simulink model "generator_trajektorie"  (R2020a)
settings: Solver=VariableStepAuto  StartTime=0.0  StopTime=Tmax  RelTol=1e-3
values from neighbouring files (symbols this model uses):
  a1 = 2    [overeniFunkcionality.m]    (also in pohyb_po_trajektorii.m; setup.m)
  a2 = 1.5    [overeniFunkcionality.m]    (also in pohyb_po_trajektorii.m; setup.m)
  a3 = 0.5    [overeniFunkcionality.m]    (also in pohyb_po_trajektorii.m; setup.m)
  r = a1-a2-a3    (= 0)    [overeniFunkcionality.m]    (also in pohyb_po_trajektorii.m; setup.m)
  R = a1+a2+a3    (= 4)    [overeniFunkcionality.m]    (also in pohyb_po_trajektorii.m; setup.m)
  T_1_0 = [cos(theta10), -sin(theta10), 0, a1*cos(theta10) ... (first row only)    [overeniFunkcionality.m]    (also in pohyb_po_trajektorii.m; setup.m)
  T_2_1 = [cos(theta20), -sin(theta20), 0, a2*cos(theta20) ... (first row only)    [overeniFunkcionality.m]    (also in pohyb_po_trajektorii.m; setup.m)
  T_3_2 = [cos(theta30), -sin(theta30), 0, a3*cos(theta30) ... (first row only)    [overeniFunkcionality.m]    (also in pohyb_po_trajektorii.m; setup.m)
  v = 0.5    [overeniFunkcionality.m]    (also in pohyb_po_trajektorii.m; setup.m)
  vmax = 1    [pohyb_po_trajektorii.m]
undefined symbols (not defined in the file or in its folder): X, Y, Z
libraries: sm_lib x56, nesl_utility x32
(part 2 of 2)

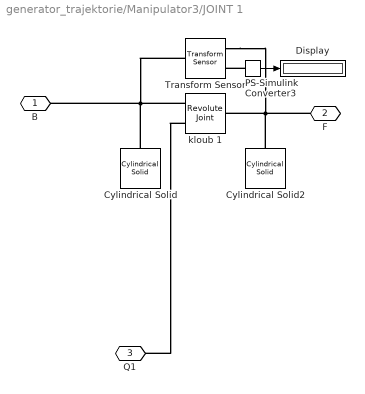
== system generator_trajektorie/Manipulator3/JOINT 1 ==
  Cylindrical Solid : sm_lib/Body Elements/Cylindrical Solid  GraphicAmbientColor=[0.15 0.15 0.15 1.0]  BasedOnType=Density  CenterOfMass=[0 0 0]  CenterOfMassUnits=m  GraphicDiffuseColor=[0.5 0.5 0.5]  CylinderLength=0.1  CylinderLengthUnits=m  CylinderRadius=0.05  CylinderRadiusUnits=m  Density=1000  DensityUnits=kg/m^3  DoExposeReferenceFrame=on  GraphicEmissiveColor=[0.0 0.0 0.0 1.0]  ExportEntireGeometry=off  SerializedFrames=<Frames/>  MarkerShape=Sphere  MarkerSize=10  GraphicType=FromGeometry  InertiaType=CalculateFromGeometry  Mass=1  MassUnits=kg  MomentsOfInertia=[1 1 1]  MomentsOfInertiaUnits=kg*m^2  GraphicOpacity=1.0  ProductsOfInertia=[0 0 0]  ProductsOfInertiaUnits=kg*m^2  GraphicShininess=75  GraphicSpecularColor=[0.5 0.5 0.5 1.0]  GraphicVisPropType=SimpleVisualProperties
  Cylindrical Solid2 : sm_lib/Body Elements/Cylindrical Solid  GraphicAmbientColor=[0.15 0.15 0.15 1.0]  BasedOnType=Density  CenterOfMass=[0 0 0]  CenterOfMassUnits=m  GraphicDiffuseColor=[0.5 0.5 0.5]  CylinderLength=0.05  CylinderLengthUnits=m  CylinderRadius=0.1  CylinderRadiusUnits=m  Density=1000  DensityUnits=kg/m^3  DoExposeReferenceFrame=on  GraphicEmissiveColor=[0.0 0.0 0.0 1.0]  ExportEntireGeometry=off  SerializedFrames=<Frames/>  MarkerShape=Sphere  MarkerSize=10  GraphicType=FromGeometry  InertiaType=CalculateFromGeometry  Mass=1  MassUnits=kg  MomentsOfInertia=[1 1 1]  MomentsOfInertiaUnits=kg*m^2  GraphicOpacity=1.0  ProductsOfInertia=[0 0 0]  ProductsOfInertiaUnits=kg*m^2  GraphicShininess=75  GraphicSpecularColor=[0.5 0.5 0.5 1.0]  GraphicVisPropType=SimpleVisualProperties
  Display : Display
  PS-Simulink Converter3 : nesl_utility/PS-Simulink Converter  PhysicalDomain=network_engine_domain  SubClassName=ps_output  LeftPortType=input  RightPortType=output  PseudoPeriodic=off  Frequencies=[]  Unit=inherit  AffineConversion=off
  Transform Sensor : sm_lib/Frames and Transforms/Transform Sensor  MeasurementFrame=Base  SenseAngle=on  SenseAxis=off  SenseAngle1=off  SenseAngle2=off  SenseAngle3=off  SenseQ=off  SenseR=off  SenseOmegaX=off  SenseOmegaY=off  SenseOmegaZ=off  SenseOmega1=off  SenseOmega2=off  SenseOmega3=off  SenseQDot=off  SenseRDot=off  SenseAlphaX=off  SenseAlphaY=off  SenseAlphaZ=off  SenseAlpha1=off  SenseAlpha2=off  SenseAlpha3=off  SenseQDDot=off  SenseRDDot=off  SenseX=off  SenseY=off  SenseZ=off  SenseRad=off  SenseAzim=off  SenseDist=off  SenseInc=off  SenseXDot=off  SenseYDot=off  SenseZDot=off  SenseRadDot=off  SenseAzimDot=off  SenseDistDot=off  SenseIncDot=off  SenseXDDot=off  SenseYDDot=off  SenseZDDot=off  SenseRadDDot=off  SenseAzimDDot=off  SenseDistDDot=off  SenseIncDDot=off
  kloub 1 : sm_lib/Joints/Revolute Joint  JointMode=Normal  SenseConstraintForce=off  SenseConstraintForceX=off  SenseConstraintForceY=off  SenseConstraintForceZ=off  SenseConstraintTorque=off  SenseConstraintTorqueX=off  SenseConstraintTorqueY=off  SenseConstraintTorqueZ=off  SenseTotalForce=off  SenseTotalForceX=off  SenseTotalForceY=off  SenseTotalForceZ=off  SenseTotalTorque=off  SenseTotalTorqueX=off  SenseTotalTorqueY=off  SenseTotalTorqueZ=off  CompositeWrenchDir=FollowerOnBase  CompositeWrenchFrame=BaseFrame  EquilibriumPosition=0  EquilibriumPositionUnits=deg  SpringStiffness=0  SpringStiffnessUnits=N*m/deg  DampingCoefficient=0  DampingCoefficientUnits=N*m/(deg/s)  TorqueActuationMode=ComputedTorque  MotionActuationMode=InputMotion  SensePosition=off  SenseVelocity=off  SenseAcceleration=off  SenseTorqueForce=off  SenseLowerLimitTorqueForce=off  SenseUpperLimitTorqueForce=off  LowerLimitSpecify=off  LowerLimitBound=-90  LowerLimitBoundUnits=deg  LowerLimitStiffness=1e4  LowerLimitStiffnessUnits=N*m/deg  LowerLimitDamping=10  LowerLimitDampingUnits=N*m/(deg/s)  LowerLimitTransitionRegionWidth=0.1  LowerLimitTransitionRegionWidthUnits=deg  UpperLimitSpecify=off  UpperLimitBound=90  UpperLimitBoundUnits=deg  UpperLimitStiffness=1e4  UpperLimitStiffnessUnits=N*m/deg  UpperLimitDamping=10  UpperLimitDampingUnits=N*m/(deg/s)  UpperLimitTransitionRegionWidth=0.1  UpperLimitTransitionRegionWidthUnits=deg  PositionTargetSpecify=off  PositionTargetPriority=High  PositionTargetValue=0  PositionTargetValueUnits=deg  VelocityTargetSpecify=off  VelocityTargetPriority=High  VelocityTargetValue=0  VelocityTargetValueUnits=deg/s
  B : PMIOPort  Side=Left
  F : PMIOPort  Port=2  Side=Right
  Q1 : PMIOPort  Port=3  Side=Left
  wires:
  PS-Simulink Converter3/1 -> Display/1
  connections:
  Cylindrical Solid2/RConn1 -- F/RConn1 -- Transform Sensor/RConn1 -- kloub 1/RConn1
  Transform Sensor/LConn1 -- B/RConn1 -- kloub 1/LConn1 -- Cylindrical Solid/RConn1
  PS-Simulink Converter3/LConn1 -- Transform Sensor/RConn2
  kloub 1/LConn2 -- Q1/RConn1

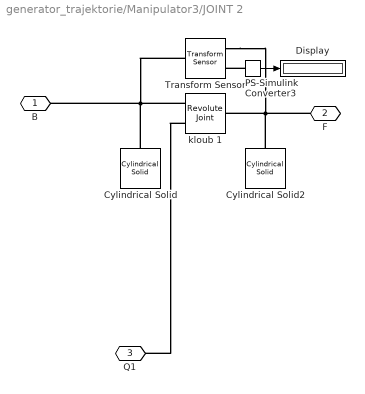
== system generator_trajektorie/Manipulator3/JOINT 2 ==
  Cylindrical Solid : sm_lib/Body Elements/Cylindrical Solid  GraphicAmbientColor=[0.15 0.15 0.15 1.0]  BasedOnType=Density  CenterOfMass=[0 0 0]  CenterOfMassUnits=m  GraphicDiffuseColor=[0.5 0.5 0.5]  CylinderLength=0.1  CylinderLengthUnits=m  CylinderRadius=0.05  CylinderRadiusUnits=m  Density=1000  DensityUnits=kg/m^3  DoExposeReferenceFrame=on  GraphicEmissiveColor=[0.0 0.0 0.0 1.0]  ExportEntireGeometry=off  SerializedFrames=<Frames/>  MarkerShape=Sphere  MarkerSize=10  GraphicType=FromGeometry  InertiaType=CalculateFromGeometry  Mass=1  MassUnits=kg  MomentsOfInertia=[1 1 1]  MomentsOfInertiaUnits=kg*m^2  GraphicOpacity=1.0  ProductsOfInertia=[0 0 0]  ProductsOfInertiaUnits=kg*m^2  GraphicShininess=75  GraphicSpecularColor=[0.5 0.5 0.5 1.0]  GraphicVisPropType=SimpleVisualProperties
  Cylindrical Solid2 : sm_lib/Body Elements/Cylindrical Solid  GraphicAmbientColor=[0.15 0.15 0.15 1.0]  BasedOnType=Density  CenterOfMass=[0 0 0]  CenterOfMassUnits=m  GraphicDiffuseColor=[0.5 0.5 0.5]  CylinderLength=0.05  CylinderLengthUnits=m  CylinderRadius=0.1  CylinderRadiusUnits=m  Density=1000  DensityUnits=kg/m^3  DoExposeReferenceFrame=on  GraphicEmissiveColor=[0.0 0.0 0.0 1.0]  ExportEntireGeometry=off  SerializedFrames=<Frames/>  MarkerShape=Sphere  MarkerSize=10  GraphicType=FromGeometry  InertiaType=CalculateFromGeometry  Mass=1  MassUnits=kg  MomentsOfInertia=[1 1 1]  MomentsOfInertiaUnits=kg*m^2  GraphicOpacity=1.0  ProductsOfInertia=[0 0 0]  ProductsOfInertiaUnits=kg*m^2  GraphicShininess=75  GraphicSpecularColor=[0.5 0.5 0.5 1.0]  GraphicVisPropType=SimpleVisualProperties
  Display : Display
  PS-Simulink Converter3 : nesl_utility/PS-Simulink Converter  PhysicalDomain=network_engine_domain  SubClassName=ps_output  LeftPortType=input  RightPortType=output  PseudoPeriodic=off  Frequencies=[]  Unit=inherit  AffineConversion=off
  Transform Sensor : sm_lib/Frames and Transforms/Transform Sensor  MeasurementFrame=Base  SenseAngle=on  SenseAxis=off  SenseAngle1=off  SenseAngle2=off  SenseAngle3=off  SenseQ=off  SenseR=off  SenseOmegaX=off  SenseOmegaY=off  SenseOmegaZ=off  SenseOmega1=off  SenseOmega2=off  SenseOmega3=off  SenseQDot=off  SenseRDot=off  SenseAlphaX=off  SenseAlphaY=off  SenseAlphaZ=off  SenseAlpha1=off  SenseAlpha2=off  SenseAlpha3=off  SenseQDDot=off  SenseRDDot=off  SenseX=off  SenseY=off  SenseZ=off  SenseRad=off  SenseAzim=off  SenseDist=off  SenseInc=off  SenseXDot=off  SenseYDot=off  SenseZDot=off  SenseRadDot=off  SenseAzimDot=off  SenseDistDot=off  SenseIncDot=off  SenseXDDot=off  SenseYDDot=off  SenseZDDot=off  SenseRadDDot=off  SenseAzimDDot=off  SenseDistDDot=off  SenseIncDDot=off
  kloub 1 : sm_lib/Joints/Revolute Joint  JointMode=Normal  SenseConstraintForce=off  SenseConstraintForceX=off  SenseConstraintForceY=off  SenseConstraintForceZ=off  SenseConstraintTorque=off  SenseConstraintTorqueX=off  SenseConstraintTorqueY=off  SenseConstraintTorqueZ=off  SenseTotalForce=off  SenseTotalForceX=off  SenseTotalForceY=off  SenseTotalForceZ=off  SenseTotalTorque=off  SenseTotalTorqueX=off  SenseTotalTorqueY=off  SenseTotalTorqueZ=off  CompositeWrenchDir=FollowerOnBase  CompositeWrenchFrame=BaseFrame  EquilibriumPosition=0  EquilibriumPositionUnits=deg  SpringStiffness=0  SpringStiffnessUnits=N*m/deg  DampingCoefficient=0  DampingCoefficientUnits=N*m/(deg/s)  TorqueActuationMode=ComputedTorque  MotionActuationMode=InputMotion  SensePosition=off  SenseVelocity=off  SenseAcceleration=off  SenseTorqueForce=off  SenseLowerLimitTorqueForce=off  SenseUpperLimitTorqueForce=off  LowerLimitSpecify=off  LowerLimitBound=-90  LowerLimitBoundUnits=deg  LowerLimitStiffness=1e4  LowerLimitStiffnessUnits=N*m/deg  LowerLimitDamping=10  LowerLimitDampingUnits=N*m/(deg/s)  LowerLimitTransitionRegionWidth=0.1  LowerLimitTransitionRegionWidthUnits=deg  UpperLimitSpecify=off  UpperLimitBound=90  UpperLimitBoundUnits=deg  UpperLimitStiffness=1e4  UpperLimitStiffnessUnits=N*m/deg  UpperLimitDamping=10  UpperLimitDampingUnits=N*m/(deg/s)  UpperLimitTransitionRegionWidth=0.1  UpperLimitTransitionRegionWidthUnits=deg  PositionTargetSpecify=off  PositionTargetPriority=High  PositionTargetValue=0  PositionTargetValueUnits=deg  VelocityTargetSpecify=off  VelocityTargetPriority=High  VelocityTargetValue=0  VelocityTargetValueUnits=deg/s
  B : PMIOPort  Side=Left
  F : PMIOPort  Port=2  Side=Right
  Q1 : PMIOPort  Port=3  Side=Left
  wires:
  PS-Simulink Converter3/1 -> Display/1
  connections:
  Transform Sensor/RConn1 -- Cylindrical Solid2/RConn1 -- kloub 1/RConn1 -- F/RConn1
  kloub 1/LConn1 -- Transform Sensor/LConn1 -- Cylindrical Solid/RConn1 -- B/RConn1
  PS-Simulink Converter3/LConn1 -- Transform Sensor/RConn2
  kloub 1/LConn2 -- Q1/RConn1

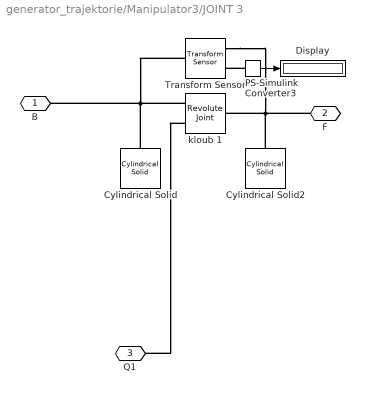
== system generator_trajektorie/Manipulator3/JOINT 3 ==
  Cylindrical Solid : sm_lib/Body Elements/Cylindrical Solid  GraphicAmbientColor=[0.15 0.15 0.15 1.0]  BasedOnType=Density  CenterOfMass=[0 0 0]  CenterOfMassUnits=m  GraphicDiffuseColor=[0.5 0.5 0.5]  CylinderLength=0.1  CylinderLengthUnits=m  CylinderRadius=0.05  CylinderRadiusUnits=m  Density=1000  DensityUnits=kg/m^3  DoExposeReferenceFrame=on  GraphicEmissiveColor=[0.0 0.0 0.0 1.0]  ExportEntireGeometry=off  SerializedFrames=<Frames/>  MarkerShape=Sphere  MarkerSize=10  GraphicType=FromGeometry  InertiaType=CalculateFromGeometry  Mass=1  MassUnits=kg  MomentsOfInertia=[1 1 1]  MomentsOfInertiaUnits=kg*m^2  GraphicOpacity=1.0  ProductsOfInertia=[0 0 0]  ProductsOfInertiaUnits=kg*m^2  GraphicShininess=75  GraphicSpecularColor=[0.5 0.5 0.5 1.0]  GraphicVisPropType=SimpleVisualProperties
  Cylindrical Solid2 : sm_lib/Body Elements/Cylindrical Solid  GraphicAmbientColor=[0.15 0.15 0.15 1.0]  BasedOnType=Density  CenterOfMass=[0 0 0]  CenterOfMassUnits=m  GraphicDiffuseColor=[0.5 0.5 0.5]  CylinderLength=0.05  CylinderLengthUnits=m  CylinderRadius=0.1  CylinderRadiusUnits=m  Density=1000  DensityUnits=kg/m^3  DoExposeReferenceFrame=on  GraphicEmissiveColor=[0.0 0.0 0.0 1.0]  ExportEntireGeometry=off  SerializedFrames=<Frames/>  MarkerShape=Sphere  MarkerSize=10  GraphicType=FromGeometry  InertiaType=CalculateFromGeometry  Mass=1  MassUnits=kg  MomentsOfInertia=[1 1 1]  MomentsOfInertiaUnits=kg*m^2  GraphicOpacity=1.0  ProductsOfInertia=[0 0 0]  ProductsOfInertiaUnits=kg*m^2  GraphicShininess=75  GraphicSpecularColor=[0.5 0.5 0.5 1.0]  GraphicVisPropType=SimpleVisualProperties
  Display : Display
  PS-Simulink Converter3 : nesl_utility/PS-Simulink Converter  PhysicalDomain=network_engine_domain  SubClassName=ps_output  LeftPortType=input  RightPortType=output  PseudoPeriodic=off  Frequencies=[]  Unit=inherit  AffineConversion=off
  Transform Sensor : sm_lib/Frames and Transforms/Transform Sensor  MeasurementFrame=Base  SenseAngle=on  SenseAxis=off  SenseAngle1=off  SenseAngle2=off  SenseAngle3=off  SenseQ=off  SenseR=off  SenseOmegaX=off  SenseOmegaY=off  SenseOmegaZ=off  SenseOmega1=off  SenseOmega2=off  SenseOmega3=off  SenseQDot=off  SenseRDot=off  SenseAlphaX=off  SenseAlphaY=off  SenseAlphaZ=off  SenseAlpha1=off  SenseAlpha2=off  SenseAlpha3=off  SenseQDDot=off  SenseRDDot=off  SenseX=off  SenseY=off  SenseZ=off  SenseRad=off  SenseAzim=off  SenseDist=off  SenseInc=off  SenseXDot=off  SenseYDot=off  SenseZDot=off  SenseRadDot=off  SenseAzimDot=off  SenseDistDot=off  SenseIncDot=off  SenseXDDot=off  SenseYDDot=off  SenseZDDot=off  SenseRadDDot=off  SenseAzimDDot=off  SenseDistDDot=off  SenseIncDDot=off
  kloub 1 : sm_lib/Joints/Revolute Joint  JointMode=Normal  SenseConstraintForce=off  SenseConstraintForceX=off  SenseConstraintForceY=off  SenseConstraintForceZ=off  SenseConstraintTorque=off  SenseConstraintTorqueX=off  SenseConstraintTorqueY=off  SenseConstraintTorqueZ=off  SenseTotalForce=off  SenseTotalForceX=off  SenseTotalForceY=off  SenseTotalForceZ=off  SenseTotalTorque=off  SenseTotalTorqueX=off  SenseTotalTorqueY=off  SenseTotalTorqueZ=off  CompositeWrenchDir=FollowerOnBase  CompositeWrenchFrame=BaseFrame  EquilibriumPosition=0  EquilibriumPositionUnits=deg  SpringStiffness=0  SpringStiffnessUnits=N*m/deg  DampingCoefficient=0  DampingCoefficientUnits=N*m/(deg/s)  TorqueActuationMode=ComputedTorque  MotionActuationMode=InputMotion  SensePosition=off  SenseVelocity=off  SenseAcceleration=off  SenseTorqueForce=off  SenseLowerLimitTorqueForce=off  SenseUpperLimitTorqueForce=off  LowerLimitSpecify=off  LowerLimitBound=-90  LowerLimitBoundUnits=deg  LowerLimitStiffness=1e4  LowerLimitStiffnessUnits=N*m/deg  LowerLimitDamping=10  LowerLimitDampingUnits=N*m/(deg/s)  LowerLimitTransitionRegionWidth=0.1  LowerLimitTransitionRegionWidthUnits=deg  UpperLimitSpecify=off  UpperLimitBound=90  UpperLimitBoundUnits=deg  UpperLimitStiffness=1e4  UpperLimitStiffnessUnits=N*m/deg  UpperLimitDamping=10  UpperLimitDampingUnits=N*m/(deg/s)  UpperLimitTransitionRegionWidth=0.1  UpperLimitTransitionRegionWidthUnits=deg  PositionTargetSpecify=off  PositionTargetPriority=High  PositionTargetValue=0  PositionTargetValueUnits=deg  VelocityTargetSpecify=off  VelocityTargetPriority=High  VelocityTargetValue=0  VelocityTargetValueUnits=deg/s
  B : PMIOPort  Side=Left
  F : PMIOPort  Port=2  Side=Right
  Q1 : PMIOPort  Port=3  Side=Left
  wires:
  PS-Simulink Converter3/1 -> Display/1
  connections:
  Transform Sensor/RConn1 -- Cylindrical Solid2/RConn1 -- kloub 1/RConn1 -- F/RConn1
  kloub 1/LConn1 -- Transform Sensor/LConn1 -- Cylindrical Solid/RConn1 -- B/RConn1
  PS-Simulink Converter3/LConn1 -- Transform Sensor/RConn2
  kloub 1/LConn2 -- Q1/RConn1

== system generator_trajektorie/Manipulator3/LINK 1 ==
  note: SUBSYSTEM RAMENE
  T_CG_1_0 : sm_lib/Frames and Transforms/Rigid Transform  TranslationMethod=Cartesian  TranslationStandardOffset=0  TranslationLengthUnit=m  TranslationStandardAxis=+Z  TranslationCartesianOffset=T_1_0(1:3,4)/2  TranslationROffset=0  TranslationROffsetUnits=m  TranslationZOffset=0  TranslationZOffsetUnits=m  TranslationThetaOffset=0  TranslationThetaOffsetUnits=deg  RotationMethod=RotationMatrix  RotationAngleUnits=deg  RotationStandardAxis=+Z  RotationAngle=0.0  RotationArbitraryAxis=[0 0 1]  FollAlignAxisA=+X  BaseAlignAxisA=+Y  FollAlignAxisB=+Y  BaseAlignAxisB=+Z  RotationSequenceAxes=FollowerAxes  RotationSequence=XYX  RotationSequenceAngles=[0 0 0]  RotationSequenceAnglesUnits=deg  RotationMatrix=T_1_0(1:3,1:3)
  Transform prvniho vuci nultymu = T_1_0 : sm_lib/Frames and Transforms/Rigid Transform  TranslationMethod=Cartesian  TranslationStandardOffset=0  TranslationLengthUnit=m  TranslationStandardAxis=+Z  TranslationCartesianOffset=T_1_0(1:3,4)  TranslationROffset=0  TranslationROffsetUnits=m  TranslationZOffset=0  TranslationZOffsetUnits=m  TranslationThetaOffset=0  TranslationThetaOffsetUnits=deg  RotationMethod=RotationMatrix  RotationAngleUnits=deg  RotationStandardAxis=+Z  RotationAngle=0.0  RotationArbitraryAxis=[0 0 1]  FollAlignAxisA=+X  BaseAlignAxisA=+Y  FollAlignAxisB=+Y  BaseAlignAxisB=+Z  RotationSequenceAxes=FollowerAxes  RotationSequence=XYX  RotationSequenceAngles=[0 0 0]  RotationSequenceAnglesUnits=deg  RotationMatrix=T_1_0(1:3,1:3)
  graficky objekt : sm_lib/Body Elements/Brick Solid  GraphicAmbientColor=[0.15 0.15 0.15 1.0]  BasedOnType=Density  BrickDimensions=[a1 0.05 0.05]  BrickDimensionUnits=m  CenterOfMass=[0 0 0]  CenterOfMassUnits=m  GraphicDiffuseColor=[0.5 0.5 0.5]  Density=1000  DensityUnits=kg/m^3  DoExposeReferenceFrame=on  GraphicEmissiveColor=[0.0 0.0 0.0 1.0]  ExportEntireGeometry=off  SerializedFrames=<Frames/>  MarkerShape=Sphere  MarkerSize=10  GraphicType=FromGeometry  InertiaType=CalculateFromGeometry  Mass=1  MassUnits=kg  MomentsOfInertia=[1 1 1]  MomentsOfInertiaUnits=kg*m^2  GraphicOpacity=1.0  ProductsOfInertia=[0 0 0]  ProductsOfInertiaUnits=kg*m^2  GraphicShininess=75  GraphicSpecularColor=[0.5 0.5 0.5 1.0]  GraphicVisPropType=SimpleVisualProperties
  CS_A : PMIOPort  Side=Left
  CS_B : PMIOPort  Port=2  Side=Right
  connections:
  Transform prvniho vuci nultymu = T_1_0/LConn1 -- CS_A/RConn1 -- T_CG_1_0/LConn1
  CS_B/RConn1 -- Transform prvniho vuci nultymu = T_1_0/RConn1
  graficky objekt/RConn1 -- T_CG_1_0/RConn1

== system generator_trajektorie/Manipulator3/LINK 2 ==
  note: SUBSYSTEM RAMENE
  T_CG_2_1 : sm_lib/Frames and Transforms/Rigid Transform  TranslationMethod=Cartesian  TranslationStandardOffset=0  TranslationLengthUnit=m  TranslationStandardAxis=+Z  TranslationCartesianOffset=T_2_1(1:3,4)/2  TranslationROffset=0  TranslationROffsetUnits=m  TranslationZOffset=0  TranslationZOffsetUnits=m  TranslationThetaOffset=0  TranslationThetaOffsetUnits=deg  RotationMethod=RotationMatrix  RotationAngleUnits=deg  RotationStandardAxis=+Z  RotationAngle=0.0  RotationArbitraryAxis=[0 0 1]  FollAlignAxisA=+X  BaseAlignAxisA=+Y  FollAlignAxisB=+Y  BaseAlignAxisB=+Z  RotationSequenceAxes=FollowerAxes  RotationSequence=XYX  RotationSequenceAngles=[0 0 0]  RotationSequenceAnglesUnits=deg  RotationMatrix=T_2_1(1:3,1:3)
  Transform druhyho vuci prvnimu = T_2_1 : sm_lib/Frames and Transforms/Rigid Transform  TranslationMethod=Cartesian  TranslationStandardOffset=0  TranslationLengthUnit=m  TranslationStandardAxis=+Z  TranslationCartesianOffset=T_2_1(1:3,4)  TranslationROffset=0  TranslationROffsetUnits=m  TranslationZOffset=0  TranslationZOffsetUnits=m  TranslationThetaOffset=0  TranslationThetaOffsetUnits=deg  RotationMethod=RotationMatrix  RotationAngleUnits=deg  RotationStandardAxis=+Z  RotationAngle=0.0  RotationArbitraryAxis=[0 0 1]  FollAlignAxisA=+X  BaseAlignAxisA=+Y  FollAlignAxisB=+Y  BaseAlignAxisB=+Z  RotationSequenceAxes=FollowerAxes  RotationSequence=XYX  RotationSequenceAngles=[0 0 0]  RotationSequenceAnglesUnits=deg  RotationMatrix=T_2_1(1:3,1:3)
  graficky objekt : sm_lib/Body Elements/Brick Solid  GraphicAmbientColor=[0.15 0.15 0.15 1.0]  BasedOnType=Density  BrickDimensions=[a2 0.05 0.05]  BrickDimensionUnits=m  CenterOfMass=[0 0 0]  CenterOfMassUnits=m  GraphicDiffuseColor=[0.5 0.5 0.5]  Density=1000  DensityUnits=kg/m^3  DoExposeReferenceFrame=on  GraphicEmissiveColor=[0.0 0.0 0.0 1.0]  ExportEntireGeometry=off  SerializedFrames=<Frames/>  MarkerShape=Sphere  MarkerSize=10  GraphicType=FromGeometry  InertiaType=CalculateFromGeometry  Mass=1  MassUnits=kg  MomentsOfInertia=[1 1 1]  MomentsOfInertiaUnits=kg*m^2  GraphicOpacity=1.0  ProductsOfInertia=[0 0 0]  ProductsOfInertiaUnits=kg*m^2  GraphicShininess=75  GraphicSpecularColor=[0.5 0.5 0.5 1.0]  GraphicVisPropType=SimpleVisualProperties
  CS_A : PMIOPort  Side=Left
  CS_B : PMIOPort  Port=2  Side=Right
  connections:
  T_CG_2_1/LConn1 -- Transform druhyho vuci prvnimu = T_2_1/LConn1 -- CS_A/RConn1
  CS_B/RConn1 -- Transform druhyho vuci prvnimu = T_2_1/RConn1
  graficky objekt/RConn1 -- T_CG_2_1/RConn1

== system generator_trajektorie/Manipulator3/LINK 3 ==
  note: SUBSYSTEM RAMENE
  T_CG_3_2 : sm_lib/Frames and Transforms/Rigid Transform  TranslationMethod=Cartesian  TranslationStandardOffset=0  TranslationLengthUnit=m  TranslationStandardAxis=+Z  TranslationCartesianOffset=T_3_2(1:3,4)/2  TranslationROffset=0  TranslationROffsetUnits=m  TranslationZOffset=0  TranslationZOffsetUnits=m  TranslationThetaOffset=0  TranslationThetaOffsetUnits=deg  RotationMethod=RotationMatrix  RotationAngleUnits=deg  RotationStandardAxis=+Z  RotationAngle=0.0  RotationArbitraryAxis=[0 0 1]  FollAlignAxisA=+X  BaseAlignAxisA=+Y  FollAlignAxisB=+Y  BaseAlignAxisB=+Z  RotationSequenceAxes=FollowerAxes  RotationSequence=XYX  RotationSequenceAngles=[0 0 0]  RotationSequenceAnglesUnits=deg  RotationMatrix=T_3_2(1:3,1:3)
  Transform tretiho vuci druhymu = T_3_2 : sm_lib/Frames and Transforms/Rigid Transform  TranslationMethod=Cartesian  TranslationStandardOffset=0  TranslationLengthUnit=m  TranslationStandardAxis=+Z  TranslationCartesianOffset=T_3_2(1:3,4)  TranslationROffset=0  TranslationROffsetUnits=m  TranslationZOffset=0  TranslationZOffsetUnits=m  TranslationThetaOffset=0  TranslationThetaOffsetUnits=deg  RotationMethod=RotationMatrix  RotationAngleUnits=deg  RotationStandardAxis=+Z  RotationAngle=0.0  RotationArbitraryAxis=[0 0 1]  FollAlignAxisA=+X  BaseAlignAxisA=+Y  FollAlignAxisB=+Y  BaseAlignAxisB=+Z  RotationSequenceAxes=FollowerAxes  RotationSequence=XYX  RotationSequenceAngles=[0 0 0]  RotationSequenceAnglesUnits=deg  RotationMatrix=T_3_2(1:3,1:3)
  graficky objekt : sm_lib/Body Elements/Brick Solid  GraphicAmbientColor=[0.15 0.15 0.15 1.0]  BasedOnType=Density  BrickDimensions=[a3 0.05 0.05]  BrickDimensionUnits=m  CenterOfMass=[0 0 0]  CenterOfMassUnits=m  GraphicDiffuseColor=[0.5 0.5 0.5]  Density=1000  DensityUnits=kg/m^3  DoExposeReferenceFrame=on  GraphicEmissiveColor=[0.0 0.0 0.0 1.0]  ExportEntireGeometry=off  SerializedFrames=<Frames/>  MarkerShape=Sphere  MarkerSize=10  GraphicType=FromGeometry  InertiaType=CalculateFromGeometry  Mass=1  MassUnits=kg  MomentsOfInertia=[1 1 1]  MomentsOfInertiaUnits=kg*m^2  GraphicOpacity=1.0  ProductsOfInertia=[0 0 0]  ProductsOfInertiaUnits=kg*m^2  GraphicShininess=75  GraphicSpecularColor=[0.5 0.5 0.5 1.0]  GraphicVisPropType=SimpleVisualProperties
  CS_A : PMIOPort  Side=Left
  CS_B : PMIOPort  Port=2  Side=Right
  connections:
  T_CG_3_2/LConn1 -- Transform tretiho vuci druhymu = T_3_2/LConn1 -- CS_A/RConn1
  CS_B/RConn1 -- Transform tretiho vuci druhymu = T_3_2/RConn1
  graficky objekt/RConn1 -- T_CG_3_2/RConn1

== matlab function generator_trajektorie/MATLAB Function2 ==
  data: x input; y input; phi input; dx input; dy input; dphi input; ddx input; ddy input; ddphi input; a1 parameter; a2 parameter; a3 parameter; theta1 output size=1; theta2 output size=1; theta3 output size=1; theta1_dot output size=1; theta2_dot output size=1; theta3_dot output size=1; theta1_dot_dot output size=1; theta2_dot_dot output size=1; theta3_dot_dot output size=1
function [theta1, theta2, theta3,theta1_dot,theta2_dot,theta3_dot,theta1_dot_dot,theta2_dot_dot,theta3_dot_dot] = IOKU( x, y, phi, dx, dy, dphi, ddx, ddy, ddphi, a1, a2, a3)

% theta2
cosQ2 = ((x - a3*cos(phi))^2 + (y - a3*sin(phi))^2 - a1^2 - a2^2)/(2 * a1 * a2);
sinQ2 = -abs(sqrt(abs(1 - cosQ2^2)));
theta2 = atan2(sinQ2, cosQ2);

% theta1
A = [-a2 * sin(theta2), a2 * cos(theta2) + a1; a2 * cos(theta2) + a1, a2 * sin(theta2)];
B = [x - a3*cos(phi); y - a3*sin(phi)];
X = A\B;
theta1 = atan2(X(1), X(2));

% theta3
theta3 = phi - theta1 - theta2;

% uhlova rychlost
JQ = [-a3 * sin(theta1 + theta2 + theta3) - a2 * sin(theta1 + theta2) - a1 * sin(theta1), -a3 * sin(theta1 + theta2 + theta3) - a2 * sin(theta1 + theta2), -a3 * sin(theta1 + theta2 + theta3);...
       a3 * cos(theta1 + theta2 + theta3) + a2 * cos(theta1 + theta2) + a1 * cos(theta1), a3 * cos(theta1 + theta2 + theta3) + a2 * cos(theta1 + theta2), a3 * cos(theta1 + theta2 + theta3);...
       1, 1, 1];
dX = [dx; dy; dphi];
dQ = JQ^(-1) * dX;
theta1_dot = dQ(1);
theta2_dot = dQ(2);
theta3_dot = dQ(3);

% uhlove zrychleni
dJQ = [-a3*cos(theta1+theta2+theta3)*(theta1_dot+theta2_dot+theta3_dot) - a2*cos(theta1+theta2)*(theta1_dot+theta2_dot) - a1*cos(theta1)*theta1_dot, -a3*cos(theta1+theta2+theta3)*(theta1_dot+theta2_dot+theta3_dot) - a2*cos(theta1+theta2)*(theta1_dot+theta2_dot), -a3*cos(theta1+theta2+theta3)*(theta1_dot+theta2_dot+theta3_dot);...
    -a3*sin(theta1+theta2+theta3)*(theta1_dot+theta2_dot+theta3_dot) - a2*sin(theta1+theta2)*(theta1_dot+theta2_dot) - a1*sin(theta1)*theta1_dot, -a3*sin(theta1+theta2+theta3)*(theta1_dot+theta2_dot+theta3_dot) - a2*sin(theta1+theta2)*(theta1_dot+theta2_dot), -a3*sin(theta1+theta2+theta3)*(theta1_dot+theta2_dot+theta3_dot);...
    0, 0, 0];
ddX = [ddx; ddy; ddphi];
ddQ = JQ^(-1) * (ddX - dJQ * dQ);
theta1_dot_dot = ddQ(1);
theta2_dot_dot = ddQ(2);
theta3_dot_dot = ddQ(3);


end

== matlab function generator_trajektorie/konstantni phi1 ==
  data: s input; Xstar output size=3; v input; a input; dXstar output size=3; ddXstar output size=3
function [Xstar, dXstar, ddXstar] = MCSstar(s, v, a)
    A = [2 0.5]';
    B = [0 1]';
%     B = [1 1]';
    C = [2 2.5]';
%     sC = -A;

    r = 0.3;
    vmax = 1;

    
    if v > vmax
        v = vmax;
    else
        v = v;
    end
    nba = (A - B)/norm(A-B);
    nbc = (C-B)/norm(C-B);
    nbs = (nba+nbc)/norm(nba+nbc);
    K1 = (nba*nba'*nbs-nbs);
    l = r/(sqrt(K1'*K1));
    S = B+nbs*l;
    k = nba'*(A-S);
    Pa = A-nba*k;
    Pc = B + norm(Pa-B)*nbc;
    
%     
%     x_pab = A-k1.*nba
    Pb = B;

    helper = (Pa-S);
    fi_pa = atan2(helper(2),helper(1));
    dir = -1;
    deltafi = acos(((Pc-S)'*(Pa-S))/r^2);
    
    s1 = norm(Pa-A);
    s2 = norm(Pc-C);
    sk = r*deltafi;
    smax = s1+s2+sk;
    if s < s1
        k1 = s;
        dk1 = v;
        ddk1 = a;
        Xstar_tmp = A-k1*nba;
        dXstar_tmp = -dk1*nba;
        ddXstar_tmp = -ddk1*nba;
    elseif s1 <= s &&  s < s1+sk
        Phi = (s-s1)/r;
        dPhi = v/r;
        ddPhi = a/r;
        
        Xstar_tmp = r* [cos(fi_pa + dir*Phi); sin(fi_pa + dir*Phi)] + S;
        dXstar_tmp = r* [-sin(fi_pa + dir*Phi); cos(fi_pa + dir*Phi)]*dir*dPhi;
        ddXstar_tmp = r* [-cos(fi_pa + dir*Phi); -sin(fi_pa + dir*Phi)]*dPhi^2 + r* [-sin(fi_pa + dir*Phi); cos(fi_pa + dir*Phi)]*dir*ddPhi;
    elseif s1+sk < s && s < s1+sk+s2
        k2 = s-s1-sk;
        dk2 = v;
        ddk2 = a;
        
        Xstar_tmp = Pc + k2*nbc;
        dXstar_tmp = dk2*nbc;
        ddXstar_tmp = ddk2*nbc;
    else
%         display('ERROR V TRAJEKTORII')
        Xstar_tmp = C;
        dXstar_tmp = zeros(2,1);
        ddXstar_tmp = zeros(2,1);
    end
    
    fi = 0;
    dfi = 0;
    ddfi = 0;

    Xstar = [Xstar_tmp; fi];
    dXstar = [dXstar_tmp; dfi];
    ddXstar = [ddXstar_tmp; ddfi];
    
   
%     
%     k1 = linspace(0,norm(A-Pa),100)
% 
% 
%     
%     fi = linspace(0,deltafi,100)
%     x_rot = [r*cos(fi_pa+dir*fi);
%              r*sin(fi_pa+dir*fi)]+S
% 
%     k2 = linspace(0,norm(Pc-C),100)
%     x_pbc = Pc + k2.*nbc
% 
% 
% 
%     smax = s1+s2+sk
%     Tmax = smax/vmax
% 
%     T = 100
%     t = linspace(0,Tmax,T)
%     t1 = linspace(0,s1/vmax,T)
%     tk = linspace(s1/vmax,sk/vmax,T)
%     t2 = linspace(sk/vmax,s2/vmax,T)
%     % s = linspace(0,smax,smax/Tmax*10)
%     s = vmax*t
% 
% 
%     k1 = 0+vmax*t
% 
%     k1 = linspace(0,s1,s1/Tmax*T)
%     fi = linspace(0,(sk)/r,(sk)/Tmax*T)
%     k2 = linspace(0,s2,s2/Tmax*T)
% 
%     
%     Xk = [r*cos(fi_pa+dir*fi);r*sin(fi_pa+dir*fi)]+S
%     X2 = Pc+k2.*nbc


end

== matlab function generator_trajektorie/MATLAB Function3 ==
  data: x input; y input; phi input; dx input; dy input; dphi input; ddx input; ddy input; ddphi input; a1 parameter; a2 parameter; a3 parameter; theta1 output size=1; theta2 output size=1; theta3 output size=1; theta1_dot output size=1; theta2_dot output size=1; theta3_dot output size=1; theta1_dot_dot output size=1; theta2_dot_dot output size=1; theta3_dot_dot output size=1
function [theta1, theta2, theta3,theta1_dot,theta2_dot,theta3_dot,theta1_dot_dot,theta2_dot_dot,theta3_dot_dot] = IOKU( x, y, phi, dx, dy, dphi, ddx, ddy, ddphi, a1, a2, a3)

% theta2
cosQ2 = ((x - a3*cos(phi))^2 + (y - a3*sin(phi))^2 - a1^2 - a2^2)/(2 * a1 * a2);
sinQ2 = -abs(sqrt(abs(1 - cosQ2^2)));
theta2 = atan2(sinQ2, cosQ2);

% theta1
A = [-a2 * sin(theta2), a2 * cos(theta2) + a1; a2 * cos(theta2) + a1, a2 * sin(theta2)];
B = [x - a3*cos(phi); y - a3*sin(phi)];
X = A\B;
theta1 = atan2(X(1), X(2));

% theta3
theta3 = phi - theta1 - theta2;

% uhlova rychlost
JQ = [-a3 * sin(theta1 + theta2 + theta3) - a2 * sin(theta1 + theta2) - a1 * sin(theta1), -a3 * sin(theta1 + theta2 + theta3) - a2 * sin(theta1 + theta2), -a3 * sin(theta1 + theta2 + theta3);...
       a3 * cos(theta1 + theta2 + theta3) + a2 * cos(theta1 + theta2) + a1 * cos(theta1), a3 * cos(theta1 + theta2 + theta3) + a2 * cos(theta1 + theta2), a3 * cos(theta1 + theta2 + theta3);...
       1, 1, 1];
dX = [dx; dy; dphi];
dQ = JQ^(-1) * dX;
theta1_dot = dQ(1);
theta2_dot = dQ(2);
theta3_dot = dQ(3);

% uhlove zrychleni
dJQ = [-a3*cos(theta1+theta2+theta3)*(theta1_dot+theta2_dot+theta3_dot) - a2*cos(theta1+theta2)*(theta1_dot+theta2_dot) - a1*cos(theta1)*theta1_dot, -a3*cos(theta1+theta2+theta3)*(theta1_dot+theta2_dot+theta3_dot) - a2*cos(theta1+theta2)*(theta1_dot+theta2_dot), -a3*cos(theta1+theta2+theta3)*(theta1_dot+theta2_dot+theta3_dot);...
    -a3*sin(theta1+theta2+theta3)*(theta1_dot+theta2_dot+theta3_dot) - a2*sin(theta1+theta2)*(theta1_dot+theta2_dot) - a1*sin(theta1)*theta1_dot, -a3*sin(theta1+theta2+theta3)*(theta1_dot+theta2_dot+theta3_dot) - a2*sin(theta1+theta2)*(theta1_dot+theta2_dot), -a3*sin(theta1+theta2+theta3)*(theta1_dot+theta2_dot+theta3_dot);...
    0, 0, 0];
ddX = [ddx; ddy; ddphi];
ddQ = JQ^(-1) * (ddX - dJQ * dQ);
theta1_dot_dot = ddQ(1);
theta2_dot_dot = ddQ(2);
theta3_dot_dot = ddQ(3);


end

== matlab function generator_trajektorie/konstantni phi2 ==
  data: s input; Xstar output size=3; v input; a input; dXstar output size=3; ddXstar output size=3
function [Xstar, dXstar, ddXstar] = MCSstar(s, v, a)
    A = [2 0.5]';
    B = [0 1]';
%     B = [1 1]';
    C = [2 2.5]';
%     sC = -A;

    r = 0.3;
    vmax = 1;

    
    if v > vmax
        v = vmax;
    else
        v = v;
    end
    nba = (A - B)/norm(A-B);
    nbc = (C-B)/norm(C-B);
    nbs = (nba+nbc)/norm(nba+nbc);
    K1 = (nba*nba'*nbs-nbs);
    l = r/(sqrt(K1'*K1));
    S = B+nbs*l;
    k = nba'*(A-S);
    Pa = A-nba*k;
    Pc = B + norm(Pa-B)*nbc;
    
%     
%     x_pab = A-k1.*nba
    Pb = B;

    helper = (Pa-S);
    fi_pa = atan2(helper(2),helper(1));
    dir = -1;
    deltafi = acos(((Pc-S)'*(Pa-S))/r^2);
    
    s1 = norm(Pa-A);
    s2 = norm(Pc-C);
    sk = r*deltafi;
    smax = s1+s2+sk;
    if s < s1
        k1 = s;
        dk1 = v;
        ddk1 = a;
        Xstar_tmp = A-k1*nba;
        dXstar_tmp = -dk1*nba;
        ddXstar_tmp = -ddk1*nba;
    elseif s1 <= s &&  s < s1+sk
        Phi = (s-s1)/r;
        dPhi = v/r;
        ddPhi = a/r;
        
        Xstar_tmp = r* [cos(fi_pa + dir*Phi); sin(fi_pa + dir*Phi)] + S;
        dXstar_tmp = r* [-sin(fi_pa + dir*Phi); cos(fi_pa + dir*Phi)]*dir*dPhi;
        ddXstar_tmp = r* [-cos(fi_pa + dir*Phi); -sin(fi_pa + dir*Phi)]*dPhi^2 + r* [-sin(fi_pa + dir*Phi); cos(fi_pa + dir*Phi)]*dir*ddPhi;
    elseif s1+sk < s && s < s1+sk+s2
        k2 = s-s1-sk;
        dk2 = v;
        ddk2 = a;
        
        Xstar_tmp = Pc + k2*nbc;
        dXstar_tmp = dk2*nbc;
        ddXstar_tmp = ddk2*nbc;
    else
%         display('ERROR V TRAJEKTORII')
        Xstar_tmp = C;
        dXstar_tmp = zeros(2,1);
        ddXstar_tmp = zeros(2,1);
    end
    
    fi = 0;
    dfi = 0;
    ddfi = 0;

    Xstar = [Xstar_tmp; fi];
    dXstar = [dXstar_tmp; dfi];
    ddXstar = [ddXstar_tmp; ddfi];
    
   
%     
%     k1 = linspace(0,norm(A-Pa),100)
% 
% 
%     
%     fi = linspace(0,deltafi,100)
%     x_rot = [r*cos(fi_pa+dir*fi);
%              r*sin(fi_pa+dir*fi)]+S
% 
%     k2 = linspace(0,norm(Pc-C),100)
%     x_pbc = Pc + k2.*nbc
% 
% 
% 
%     smax = s1+s2+sk
%     Tmax = smax/vmax
% 
%     T = 100
%     t = linspace(0,Tmax,T)
%     t1 = linspace(0,s1/vmax,T)
%     tk = linspace(s1/vmax,sk/vmax,T)
%     t2 = linspace(sk/vmax,s2/vmax,T)
%     % s = linspace(0,smax,smax/Tmax*10)
%     s = vmax*t
% 
% 
%     k1 = 0+vmax*t
% 
%     k1 = linspace(0,s1,s1/Tmax*T)
%     fi = linspace(0,(sk)/r,(sk)/Tmax*T)
%     k2 = linspace(0,s2,s2/Tmax*T)
% 
%     
%     Xk = [r*cos(fi_pa+dir*fi);r*sin(fi_pa+dir*fi)]+S
%     X2 = Pc+k2.*nbc


end
